simulink model "SeparatelyExcitedDCMotorModelling"  (R2018a)
settings: Solver=VariableStepAuto  StartTime=0.0  StopTime=10  RelTol=1e-3
settings Model: Creator=Neo  LastModifiedBy=Neo

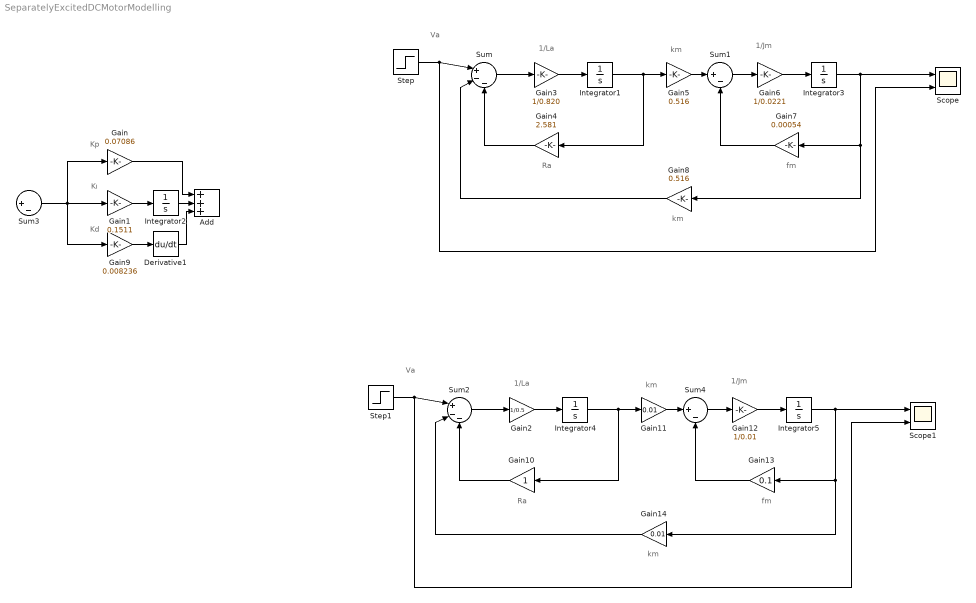
== system SeparatelyExcitedDCMotorModelling ==
  note: km
  note: fm
  note: Kı
  note: km
  note: Kp
  note: 1/Jm
  note: Kd
  note: Va
  note: Ra
  note: 1/La
  note: Ra
  note: Va
  note: 1/La
  note: km
  note: fm
  note: km
  note: 1/Jm
  Add : Sum  Inputs=+++
  Derivative1 : Derivative
  Gain : Gain  Gain=0.07086
  Gain1 : Gain  Gain=0.1511
  Gain10 : Gain
  Gain11 : Gain  Gain=0.01
  Gain12 : Gain  Gain=1/0.01
  Gain13 : Gain  Gain=0.1
  Gain14 : Gain  Gain=0.01
  Gain2 : Gain  Gain=1/0.5
  Gain3 : Gain  Gain=1/0.820
  Gain4 : Gain  Gain=2.581
  Gain5 : Gain  Gain=0.516
  Gain6 : Gain  Gain=1/0.0221
  Gain7 : Gain  Gain=0.00054
  Gain8 : Gain  Gain=0.516
  Gain9 : Gain  Gain=0.008236
  Integrator{1..5} (5 alike) : Integrator
  Scope : Scope  NumInputPorts=2
  Scope1 : Scope  NumInputPorts=2
  Step : Step  Time=0  After=100  SampleTime=0
  Step1 : Step  Time=0  After=10  SampleTime=0
  Sum : Sum  Inputs=|+--
  Sum1 : Sum  Inputs=|+-
  Sum2 : Sum  Inputs=|+--
  Sum3 : Sum  Inputs=|+-
  Sum4 : Sum  Inputs=|+-
  wires:
  Gain5/1 -> Sum1/1
  Sum3/1 -> Gain/1, Gain9/1, Gain1/1
  Integrator2/1 -> Add/2
  Integrator3/1 -> Gain8/1, Gain7/1, Scope/1
  Step/1 -> Sum/1, Scope/2
  Sum/1 -> Gain3/1
  Gain1/1 -> Integrator2/1
  Gain9/1 -> Derivative1/1
  Gain/1 -> Add/1
  Gain7/1 -> Sum1/2
  Sum1/1 -> Gain6/1
  Derivative1/1 -> Add/3
  Gain3/1 -> Integrator1/1
  Integrator1/1 -> Gain5/1, Gain4/1
  Gain6/1 -> Integrator3/1
  Gain4/1 -> Sum/3
  Gain8/1 -> Sum/2
  Gain13/1 -> Sum4/2
  Integrator5/1 -> Gain14/1, Gain13/1, Scope1/1
  Sum2/1 -> Gain2/1
  Gain10/1 -> Sum2/3
  Gain11/1 -> Sum4/1
  Gain12/1 -> Integrator5/1
  Gain2/1 -> Integrator4/1
  Integrator4/1 -> Gain11/1, Gain10/1
  Sum4/1 -> Gain12/1
  Step1/1 -> Sum2/1, Scope1/2
  Gain14/1 -> Sum2/2
